simulink model "week1problem5"  (R2020b)
settings: Solver=VariableStepAuto  StartTime=0.0  StopTime=10.0  RelTol=1e-3
undefined symbols (not defined in the file): C, R
settings Model: Creator=Puru Gawande  LastModifiedBy=Puru Gawande

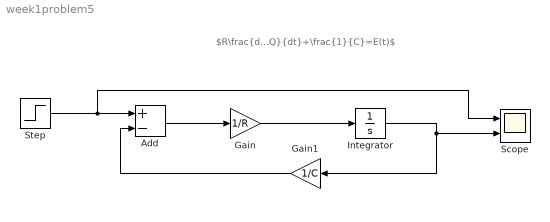
== system week1problem5 ==
  note: $R\frac{dQ}{dt}+\frac{1}{C}=E(t)$
  Add : Sum  Inputs=+-
  Gain : Gain  Gain=1/R
  Gain1 : Gain  Gain=1/C
  Integrator : Integrator  InitialCondition=8
  Scope : Scope  NumInputPorts=2
  Step : Step  Before=1  After=3  SampleTime=0
  wires:
  Step/1 -> Scope/1, Add/1
  Add/1 -> Gain/1
  Gain/1 -> Integrator/1
  Integrator/1 -> Gain1/1, Scope/2
  Gain1/1 -> Add/2
